simulink model "lftModel"  (R2024a)
settings: Solver=ode1  StartTime=0.0  StopTime=Inf  FixedStep=0.001  RelTol=1e-3
PostLoadFcn:
  | , if any(exist('dsrtsu_mdlpostloadfcn', 'file') ~= 0), dsrtsu_mdlpostloadfcn('Execute', bdroot); end,
InitFcn:
  | , if any(exist('rtifpga_mdlclblib', 'file') ~= 0), rtifpga_mdlclblib('Init', bdroot); end,
undefined symbols (not defined in the file): ampN, Current_Limit, cycles, fb, ff, fHz, fIN, freqs, lc, lcam, Mag_xData, Mag_yData, trajData, wn, xData, yData, z_stroke, z_TDC
libraries: rti1202lib_adc_class1 x7, rti1202lib_dio_class1 x3, simulink x3, rti1202lib_dac_class1 x1
(part 3 of 4)

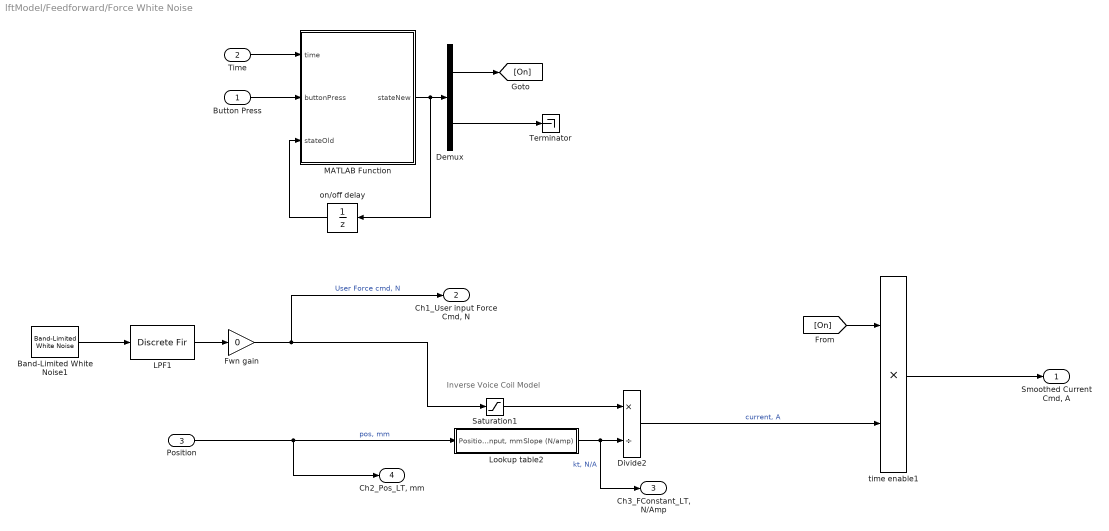
== system lftModel/Feedforward/Force White Noise  ==
  note: Inverse Voice Coil Model
  Button Press : Inport
  Time : Inport  Port=2
  Position : Inport  Port=3
  Band-Limited White Noise1 : simulink/Sources/Band-Limited White Noise  Cov=[.1]  Ts=1e-3  seed=[23341]
  Demux : Demux  Outputs=2
  Divide2 : Product  Inputs=*/
  Fwn gain : Gain  Gain=0
  LPF1 : DiscreteFir  Tag=BlockMethodSubSystem  Coefficients=[0.00631128081582466201 0.00013543430278497223 0.000136870196923014959 0.000138307894980391801 0.000139745838967405081 0.000141180859676371512 0.000142612008190714297 0.000144041366817015644 0.000145467420040382801 0.000146886341234289024 0.000148298674128573299 0.00014970828980578161 0.000151105462927332546 0.000152485453613127584 0.000153856505328838031 0.000155204886984408868 0.000156537614709266232 0.000157844715122636755 0.000159126589617151863 0.000160377867746102688 0.00016159347907830827 0.000162771425864857299 0.00016391074233170329 0.000165008373666045578 0.000166060320108453869 0.000167070411019297574 0.000168031314016722229 0.000168957010872338147 0.000169840775091942709 0.000170702427809726751 0.000171556051355427108 0.000172411492316374679 0.000173297144485036448 0.000174248500430531408 0.000175305359989292827 0.000176519392725154489 0.000177960129667976372 0.00017971114900722663 0.000181871119101426754 0.000184559719422111042 0.000176105661326144477 0.000181749708229284149 0.000182466858202373665 0.000183157791520970168 0.000183822446350530419 0.000184463684187331409 0.0001850836021499301 0.000185680317358461854 0.000186254166863032271 0.000186808631915639394 0.000187343119584809203 0.000187849842539686778 0.000188334426245146509 0.000188801168286149309 0.00018923837437738133 0.000189655003001403433 0.000190039581192655635 0.000190395398476439341 0.000190715906213227146 0.000190999304257855393 0.000191245064733318819 0.000191450307200052389 0.000191610753881228159 0.000191724878321957885 0.000191795437400793295 0.000191818465477217194 0.000191808015455337819 0.000191757656910983157 0.000191690685709788161 0.000191607502262395625 0.000191515276584489373 0.00019143355495045768 0.00019136780431717074 0.000191313757509944937 0.000191257961261410059 0.000191164264085296614 0.000190954162439371702 0.000190493576723921976 0.000189572245447842735 0.000187870706712464701 0.0001897339034343202 0.000188385981482907269 0.000187843264996656844 0.000187260723632739226 0.000186640674608572307 0.000185982434791956137 0.00018528449737709323 0.000184549288945726067 0.00018377798356300563 0.000182967304729899 0.000182115987315683366 0.000181232639653812396 0.000180313291305732906 0.000179350381237631656 0.000178352306006916911 0.00017730705711621142 0.000176220778563580024 0.000175086212295391441 0.000173904918410652251 0.000172675148258410576 0.000171393159966842876 0.000170057676525047966 0.000168671270477623465 0.000167237213232533557 0.000165756225529311674 0.000164241060646810655 0.000162686086082531423 0.000161111925583595035 0.000159506378329737127 0.000157878499974526998 0.000156232100918046236 0.000154549063579370556 0.00015281149649245114 0.000150998724147295764 0.000149083264485818713 0.000147043764881427531 0.000144896207155866018 0.000142732405000378789 0.000140782991689901389 0.000139522446253002673 0.00013645475112169264 0.000134500458434938627 0.00013225075613465954 0.000129957455551248731 0.000127618920583867027 0.000125235867550077936 0.000122811014255850176 0.000120343372162943566 0.000117831796564274764 0.000115279950352218191 0.000112691550200662085 0.000110057341665872034 0.000107376984638812145 0.000104656167138775309 0.000101884038473241874 9.90686359278970731e-05 9.62016020808731501e-05 9.32866927548676452e-05 9.03202184661189094e-05 8.73012222788652323e-05 8.42331104386443319e-05 8.11202454982114365e-05 7.79653006870085526e-05 7.4771163122194266e-05 7.15458567965872175e-05 6.82827144445772238e-05 6.49954777320802646e-05 6.16643478750626705e-05 5.8301185783228919e-05 5.48930965835259512e-05 5.14200931737376655e-05 4.78794300989164972e-05 4.42697147388638166e-05 4.05958948104637827e-05 3.68834441127705652e-05 3.31795820304337251e-05 2.95277219982310551e-05 2.59163554410707452e-05 2.21704322481949188e-05 1.77345612084081143e-05 1.42389535967590552e-05 1.01907533750498876e-05 6.1946549781969285e-06 2.15703917919321561e-06 -1.91931685908737764e-06 -6.03280379512105157e-06 -1.01845904286679383e-05 ...(+30067 chars)]  InputProcessing=Columns as channels (frame based)
  Lookup table2 : Subsystem
  MATLAB Function : MATLAB Function  TreatAsAtomicUnit=on
  Saturation1 : Saturate  UpperLimit=fIN.Forcemax  LowerLimit=-fIN.Forcemax
  Terminator : Terminator
  on/off delay : UnitDelay  InitialCondition=[0, 0]  SampleTime=-1  HasFrameUpgradeWarning=on
      settings: AttributesFormatString=IC: %<X0>
  time enable1 : Product  Inputs=**
  "Smoothed Current Cmd, A" : Outport
  "Ch1_User input Force Cmd, N" : Outport  Port=2
  "Ch3_FConstant_LT, N/Amp" : Outport  Port=3
  "Ch2_Pos_LT, mm" : Outport  Port=4
  wires:
  on/off delay/1 -> MATLAB Function/3(stateOld)
  Button Press/1 -> MATLAB Function/2(buttonPress)
  Time/1 -> MATLAB Function/1(time)
  MATLAB Function/1(stateNew) -> on/off delay/1, Demux/1
  Demux/1 -> [On]
  Demux/2 -> Terminator/1
  [On] -> time enable1/1
  Lookup table2/1(Slope (N/amp)) -> "Ch3_FConstant_LT, N/Amp"/1, Divide2/2  "kt, N/A"
  Divide2/1 -> time enable1/2  "current, A"
  Saturation1/1 -> Divide2/1
  time enable1/1 -> "Smoothed Current Cmd, A"/1
  Position/1 -> "Ch2_Pos_LT, mm"/1, Lookup table2/1("Position Input, mm")  "pos, mm"
  LPF1/1 -> Fwn gain/1
  Band-Limited White Noise1/1 -> LPF1/1
  Fwn gain/1 -> Saturation1/1, "Ch1_User input Force Cmd, N"/1  "User Force cmd, N"

== system lftModel/Feedforward/Sine Wave ==
  Button Press : Inport
  Time : Inport  Port=2
  MATLAB Function : MATLAB Function  TreatAsAtomicUnit=on
  unit delay : UnitDelay  InitialCondition=[0, 0]  SampleTime=-1  HasFrameUpgradeWarning=on
      settings: AttributesFormatString=IC: %<X0>
  "Smoothed Current Cmd, A" : Outport
  wires:
  Time/1 -> MATLAB Function/2(time)
  Button Press/1 -> MATLAB Function/1(buttonPress)
  unit delay/1 -> MATLAB Function/3(stateOld)
  MATLAB Function/1(yOut) -> "Smoothed Current Cmd, A"/1  "cmd"
  MATLAB Function/2(stateNew) -> unit delay/1

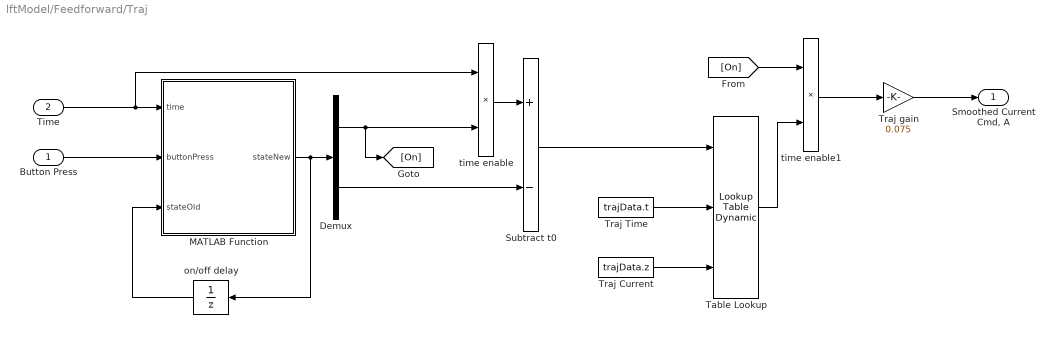
== system lftModel/Feedforward/Traj ==
  Button Press : Inport
  Time : Inport  Port=2
  Demux : Demux  Outputs=2
  MATLAB Function : MATLAB Function  TreatAsAtomicUnit=on
  Subtract t0 : Sum  Inputs=+-
  Table Lookup : simulink/Lookup Tables/Lookup Table Dynamic  LookUpMeth=Interpolation-Use End Values  OutDataType=fixdt('double')  OutScaling=[]  OutputDataTypeScalingMode=Specify via dialog  OutDataTypeStr=double  DoSatur=off
  Traj Current : Constant  Value=trajData.z
  Traj Time : Constant  Value=trajData.t
  Traj gain : Gain  Gain=0.075
  on/off delay : UnitDelay  InitialCondition=[0, 0]  SampleTime=-1  HasFrameUpgradeWarning=on
      settings: AttributesFormatString=IC: %<X0>
  time enable : Product  Inputs=**
  time enable1 : Product  Inputs=**
  "Smoothed Current Cmd, A" : Outport
  wires:
  Traj gain/1 -> "Smoothed Current Cmd, A"/1
  time enable1/1 -> Traj gain/1
  [On] -> time enable1/1
  Demux/2 -> Subtract t0/2
  Demux/1 -> time enable/2, [On]
  time enable/1 -> Subtract t0/1
  MATLAB Function/1(stateNew) -> Demux/1, on/off delay/1
  Traj Current/1 -> Table Lookup/3
  Traj Time/1 -> Table Lookup/2
  Table Lookup/1 -> time enable1/2
  Subtract t0/1 -> Table Lookup/1
  Time/1 -> MATLAB Function/1(time), time enable/1
  Button Press/1 -> MATLAB Function/2(buttonPress)
  on/off delay/1 -> MATLAB Function/3(stateOld)

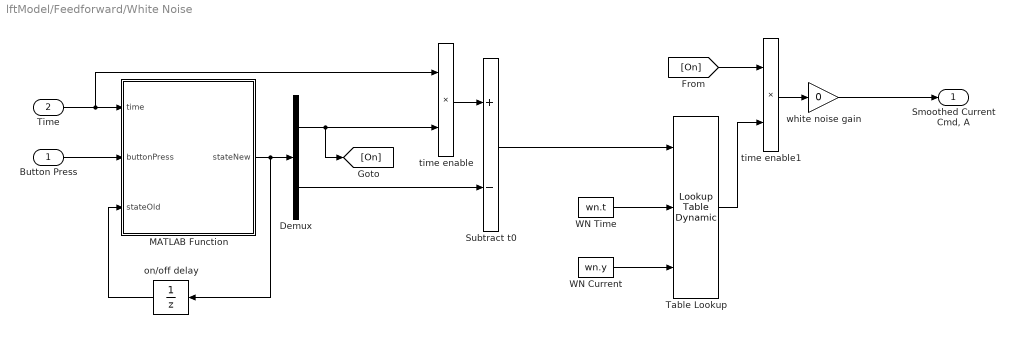
== system lftModel/Feedforward/White Noise ==
  Button Press : Inport
  Time : Inport  Port=2
  Demux : Demux  Outputs=2
  MATLAB Function : MATLAB Function  TreatAsAtomicUnit=on
  Subtract t0 : Sum  Inputs=+-
  Table Lookup : simulink/Lookup Tables/Lookup Table Dynamic  LookUpMeth=Interpolation-Use End Values  OutDataType=fixdt('double')  OutScaling=[]  OutputDataTypeScalingMode=Specify via dialog  OutDataTypeStr=double  DoSatur=off
  WN Current : Constant  Value=wn.y
  WN Time : Constant  Value=wn.t
  on/off delay : UnitDelay  InitialCondition=[0, 0]  SampleTime=-1  HasFrameUpgradeWarning=on
      settings: AttributesFormatString=IC: %<X0>
  time enable : Product  Inputs=**
  time enable1 : Product  Inputs=**
  white noise gain : Gain  Gain=0
  "Smoothed Current Cmd, A" : Outport
  wires:
  on/off delay/1 -> MATLAB Function/3(stateOld)
  Button Press/1 -> MATLAB Function/2(buttonPress)
  Time/1 -> time enable/1, MATLAB Function/1(time)
  Subtract t0/1 -> Table Lookup/1
  Table Lookup/1 -> time enable1/2
  WN Time/1 -> Table Lookup/2
  WN Current/1 -> Table Lookup/3
  MATLAB Function/1(stateNew) -> on/off delay/1, Demux/1
  time enable/1 -> Subtract t0/1
  Demux/1 -> [On], time enable/2
  Demux/2 -> Subtract t0/2
  [On] -> time enable1/1
  time enable1/1 -> white noise gain/1
  white noise gain/1 -> "Smoothed Current Cmd, A"/1

== system lftModel/Feedforward/Zero ==
  Button Press : Inport
  Time : Inport  Port=2
  Constant : Constant  Value=0
  Terminator : Terminator
  "Smoothed Current Cmd, A" : Outport
  wires:
  Button Press/1 -> Terminator/1
  Constant/1 -> "Smoothed Current Cmd, A"/1

== system lftModel/Magnetic field cancellation/Look up-Meg ==
  pos : Inport
  Lookup with Linear Lagrange Interpolation1 : Lookup_n-D  NumberOfTableDimensions=1  BreakpointsForDimension1=Mag_xData  Table=Mag_yData  InterpMethod=Linear Lagrange  InternalRulePriority=Speed  RndMeth=Simplest
  "Force meg, N" : Outport
  wires:
  pos/1 -> Lookup with Linear Lagrange Interpolation1/1
  Lookup with Linear Lagrange Interpolation1/1 -> "Force meg, N"/1

== system lftModel/Magnetic field cancellation/Lookup - Slope ==
  "Position Input, mm" : Inport
  Lookup with Linear Lagrange Interpolation : Lookup_n-D  NumberOfTableDimensions=1  BreakpointsForDimension1=xData  Table=yData  InterpMethod=Linear Lagrange  InternalRulePriority=Speed  RndMeth=Simplest
  Slope (N/amp) : Outport
  wires:
  "Position Input, mm"/1 -> Lookup with Linear Lagrange Interpolation/1
  Lookup with Linear Lagrange Interpolation/1 -> Slope (N/amp)/1

== system lftModel/RTI Data/RTI Data Store ==
  RTI Data Store : Subsystem  mask(RTI_DATA_STORE){}
      mask help:
      | RTI Data Store Block. This block is used by RTI to store internal model dependent data. Deleting this block will result in data loss.
      |
      | NEVER DELETE, COPY, OR MODIFY THIS BLOCK!
      mask Help:
      | RTI Data Store Block. This block is used by RTI to store internal model dependent data. Deleting this block will result in data loss.
      | 
      | NEVER DELETE, COPY, OR MODIFY THIS BLOCK!
      mask Display: text(0.5, 0.5, ' ', 'HorizontalAlignment', 'center');

== system lftModel/Sweep Test/Subsystem1 ==
  note: Inverse Voice Coil Model
  Position : Inport
  Sweep Force Input : Inport  Port=2
  Divide2 : Product  Inputs=*/
  Lookup table2 : Subsystem
  Saturation1 : Saturate  UpperLimit=fIN.Forcemax  LowerLimit=-fIN.Forcemax
  "Sweep Force Cmd, N" : Outport
  "Current, A" : Outport  Port=2
  "Ch2_Pos_LT, mm1" : Outport  Port=3
  wires:
  Sweep Force Input/1 -> "Sweep Force Cmd, N"/1, Saturation1/1  "Total Force cmd, N"
  Lookup table2/1(Slope (N/amp)) -> Divide2/2  "kt, N/A"
  Position/1 -> "Ch2_Pos_LT, mm1"/1, Lookup table2/1("Position Input, mm")
  Saturation1/1 -> Divide2/1
  Divide2/1 -> "Current, A"/1  "Current, A"

== system lftModel/Feedbackward Current/Damping Feedback/Lookup table2 ==
  "Position Input, mm" : Inport
  Lookup with Linear Lagrange Interpolation : Lookup_n-D  NumberOfTableDimensions=1  BreakpointsForDimension1=xData  Table=yData  InterpMethod=Linear Lagrange  InternalRulePriority=Speed  RndMeth=Simplest
  Slope (N/amp) : Outport
  wires:
  Lookup with Linear Lagrange Interpolation/1 -> Slope (N/amp)/1
  "Position Input, mm"/1 -> Lookup with Linear Lagrange Interpolation/1

== system lftModel/Feedforward/FConstant/Lookup - Slope ==
  "Position Input, mm" : Inport
  Lookup with Linear Lagrange Interpolation : Lookup_n-D  NumberOfTableDimensions=1  BreakpointsForDimension1=xData  Table=yData  InterpMethod=Linear Lagrange  InternalRulePriority=Speed  RndMeth=Simplest
  Slope (N/amp) : Outport
  wires:
  Lookup with Linear Lagrange Interpolation/1 -> Slope (N/amp)/1
  "Position Input, mm"/1 -> Lookup with Linear Lagrange Interpolation/1

== system lftModel/Feedforward/FTraj /Lookup table2 ==
  "Position Input, mm" : Inport
  Lookup with Linear Lagrange Interpolation : Lookup_n-D  NumberOfTableDimensions=1  BreakpointsForDimension1=xData  Table=yData  InterpMethod=Linear Lagrange  InternalRulePriority=Speed  RndMeth=Simplest
  Slope (N/amp) : Outport
  wires:
  Lookup with Linear Lagrange Interpolation/1 -> Slope (N/amp)/1
  "Position Input, mm"/1 -> Lookup with Linear Lagrange Interpolation/1

== system lftModel/Feedforward/Force White Noise /Lookup table2 ==
  "Position Input, mm" : Inport
  Lookup with Linear Lagrange Interpolation : Lookup_n-D  NumberOfTableDimensions=1  BreakpointsForDimension1=xData  Table=yData  InterpMethod=Linear Lagrange  InternalRulePriority=Speed  RndMeth=Simplest
  Slope (N/amp) : Outport
  wires:
  Lookup with Linear Lagrange Interpolation/1 -> Slope (N/amp)/1
  "Position Input, mm"/1 -> Lookup with Linear Lagrange Interpolation/1

== system lftModel/RTI Data/RTI Data Store/RTI Data Store ==
  RTI Data Store : Subsystem  mask(RTI_DATA_STORE){}
      mask help:
      | RTI Data Store Block. This block is used by RTI to store internal model dependent data. Deleting this block will result in data loss.
      |
      | NEVER DELETE, COPY, OR MODIFY THIS BLOCK!
      mask Help:
      | RTI Data Store Block. This block is used by RTI to store internal model dependent data. Deleting this block will result in data loss.
      | 
      | NEVER DELETE, COPY, OR MODIFY THIS BLOCK!
      mask Display: text(0.5, 0.5, ' ', 'HorizontalAlignment', 'center');

== system lftModel/Sweep Test/Subsystem1/Lookup table2 ==
  "Position Input, mm" : Inport
  Lookup with Linear Lagrange Interpolation : Lookup_n-D  NumberOfTableDimensions=1  BreakpointsForDimension1=xData  Table=yData  InterpMethod=Linear Lagrange  InternalRulePriority=Speed  RndMeth=Simplest
  Slope (N/amp) : Outport
  wires:
  Lookup with Linear Lagrange Interpolation/1 -> Slope (N/amp)/1
  "Position Input, mm"/1 -> Lookup with Linear Lagrange Interpolation/1

== system lftModel/RTI Data/RTI Data Store/RTI Data Store/RTI Data Store ==
  RTI Data Store : Subsystem  mask(RTI_DATA_STORE){}
      mask help:
      | RTI Data Store Block. This block is used by RTI to store internal model dependent data. Deleting this block will result in data loss.
      |
      | NEVER DELETE, COPY, OR MODIFY THIS BLOCK!
      mask Help:
      | RTI Data Store Block. This block is used by RTI to store internal model dependent data. Deleting this block will result in data loss.
      | 
      | NEVER DELETE, COPY, OR MODIFY THIS BLOCK!
      mask Display: text(0.5, 0.5, ' ', 'HorizontalAlignment', 'center');

== system lftModel/RTI Data/RTI Data Store/RTI Data Store/RTI Data Store/RTI Data Store ==

== matlab function lftModel/Feedforward/White Noise/MATLAB Function ==
  data: time input size=1; buttonPress input size=1; stateOld input size=2; stateNew output size=2
function stateNew = onoffToggle(time,buttonPress,stateOld)
% ONOFFTOGGLE starts a sine wave when buttonPress goes high and turns it off
% when it goes low
%
% If the sine wave playState is OFF when the button is pressed, then the
% current time is latched, and the sine wave is started. If the button is
% pressed when the sine wave playState is ON, then time is reset to zero
% and the sine wave stops immediately.
%
% Truth table
%   buttonPress      playState     Action
%  ------------------------------------------------------------------------
%       0                0         timeState = 0
%                                  playState = 0
%                                  yOut = 0
%       0                1         timeState = 0
%                                  playState = 0
%                                  yOut = 0
%       1                0         timeState = time
%                                  playState = 1
%                                  yOut = sine(time-timeState)
%       1                1         timeState = no change
%                                  playState = no change
%                                  yOut = sine(time-timeState)

  % Set buttonPress to 0 or 1 despite what any user tries to do...
  if buttonPress < 0
      buttonPress = 0;
  end

  if buttonPress > 1
      buttonPress = 1;
  end

  % Extract a states
  timeStateOld = stateOld(2);
  playStateOld = stateOld(1);  

  % Init, default the output = 0, and the new states = old states
  timeStateNew = timeStateOld;
  playStateNew = playStateOld;

  % Implement truth table
  if ~buttonPress
      timeStateNew = 0;
      playStateNew = 0;
  elseif ~playStateOld
      timeStateNew = time;
      playStateNew = 1;
  end

  % Update state
  stateNew = [playStateNew; timeStateNew];
